simulink model "sedemo_shared_access_media"  (Simulink 7.5)
settings: Solver=VariableStepDiscrete  StartTime=0.0  StopTime=300  MaxStep=inf  RelTol=1e-3
undefined symbols (not defined in the file or in its folder): des_attributefunction_support, slcm
libraries: simeventsattributes2 x7, simeventssink1 x7, simeventsgenerators1 x5, simulink x4, simeventsrouting1 x4, simeventsqueue1 x3, simeventstranslate1 x1, simeventssignalmanage1 x1, simeventsserver1 x1
settings Model: DataTypeOverride=TrueDoubles  MinMaxOverflowLogging=ForceOff  Creator=The MathWorks Inc.  ExtModeAutoUpdateStatusClock=off
settings DataIOCC: SaveOutput=off  SaveTime=off
settings OptimizationCC: InlineInvariantSignals=on  InitFltsAndDblsToZero=on
settings DebuggingCC: AlgebraicLoopMsg=error  SaveWithParameterizedLinksMsg=none  SignalResolutionControl=TryResolveAllWithWarning  SolverPrmCheckMsg=none  InheritedTsInSrcMsg=none  DiscreteInheritContinuousMsg=none  MultiTaskDSMMsg=warning  MultiTaskCondExecSysMsg=none  StrictBusMsg=None
settings RTWCC: IncludeERTFirstTime=on
settings GRTTargetCC: TargetFcnLib=ansi_tfl_tmw.mat
settings SimEventsCC: propIdentEventSeed=12345678  propDiagAttribOutput=1  propDiagFcnCallOutput=1  propDiagStatOutput=0

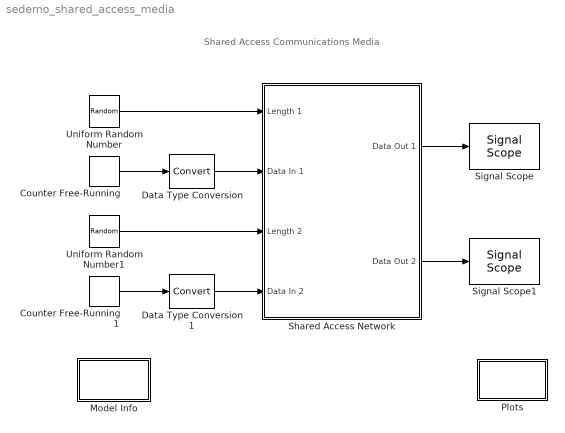
== system sedemo_shared_access_media ==
  note: Shared Access Communications Media
  Counter Free-Running : simulink/Sources/Counter Free-Running  SystemSampleTime=-1  NumBits=20  tsamp=-1
  Counter Free-Running1 : simulink/Sources/Counter Free-Running  SystemSampleTime=-1  NumBits=20  tsamp=-1
  Data Type Conversion : DataTypeConversion  OutDataType=sfix(16)  OutScaling=2^0
  Data Type Conversion1 : DataTypeConversion  OutDataType=sfix(16)  OutScaling=2^0
  Model Info : Subsystem  LoadFcn=slcm LoadBlock;  InitFcn=slcm('UpdateAllCMBlocksInThisModelInit')  mask(CMBlock){InitialSaveTempField=, InitialBlockCM=None, BlockCM=None, Frame=on, SaveTempField=, DisplayStringWithTags=Info, MaskDisplayString=Info, HorizontalTextAlignment=Center, LeftAlignmentValue=0.5, SourceBlockDiagram=sedemo_shared_access_media, TagMaxNumber=20, CMTag1=, CMTag2=, CMTag3=, CMTag4=, CMTag5=, CMTag6=, CMTag7=, CMTag8=, CMTag9=, CMTag10=, CMTag11=, CMTag12=, CMTag13=, CMTag14=, CMTag15=, CMTag16=, CMTag17=, CMTag18=, CMTag19=, CMTag20=}
      mask help: This block allows revision control information to be displayed within the model.
      settings: CopyFcn=slcm CopyBlock;  DeleteFcn=slcm Cancel;  PostSaveFcn=slcm('UpdateAllCMBlocksInThisModel')  NameChangeFcn=slcm Rename;  OpenFcn=open_system([gcb '/Information'])
      mask Display: text(str2num(LeftAlignmentValue), 0.5, MaskDisplayString, 'HorizontalAlignment', HorizontalTextAlignment)
  Plots : Subsystem
      settings: RequestExecContextInheritance=on
  Shared Access Network : Subsystem
  Signal Scope : simeventssink1/Signal Scope  Priority=1  SystemSampleTime=-1  PlotType=Stem  InputType=Signal  NumInputs=1  AttributeNameY=Count  XInputOptionSignal=Event time  XInputOptionEntity=Event time  AttributeNameX=Count  EnableEntityOutport=on  XMin=0  XMax=10  XLimitExceededOption=Stretch axis limits  YLimitExceededOption=Stretch axis limits  AxisGrid=on  AxisLegend=off  LineDisables=""  LineColors=b  LineStyles=-  LineMarkers=.  OpenScopeAtSimStart=off  Title=Data Value at Destination 1  YLabel=Data Value  XLabel=Time  FigurePosition=[4 747 305 208]  AxisZoom=off  DataStoreOption=Limited  DataPointsLimit=10000  StatNumberArrived=Off  ShowCountPlotted=on  ShowToolbar=on
      settings: YMin=0  YMax=10
  Signal Scope1 : simeventssink1/Signal Scope  Priority=1  SystemSampleTime=-1  PlotType=Stem  InputType=Signal  NumInputs=1  AttributeNameY=Count  XInputOptionSignal=Event time  XInputOptionEntity=Event time  AttributeNameX=Count  EnableEntityOutport=on  XMin=0  XMax=10  XLimitExceededOption=Stretch axis limits  YLimitExceededOption=Stretch axis limits  AxisGrid=on  AxisLegend=off  LineDisables=""  LineColors=b  LineStyles=-  LineMarkers=.  OpenScopeAtSimStart=off  Title=Data Value at Destination 1  YLabel=Data Value  XLabel=Time  FigurePosition=[4 465 305 208]  AxisZoom=off  DataStoreOption=Limited  DataPointsLimit=10000  StatNumberArrived=Off  ShowCountPlotted=on  ShowToolbar=on
      settings: YMin=0  YMax=10
  Uniform Random Number : UniformRandomNumber  Minimum=20  Maximum=2000  Seed=12345  SampleTime=0
  Uniform Random Number1 : UniformRandomNumber  Minimum=20  Maximum=2000  Seed=234567  SampleTime=0
  wires:
  Uniform Random Number/1 -> Shared Access Network/1(Length 1)
  Counter Free-Running/1 -> Data Type Conversion/1
  Uniform Random Number1/1 -> Shared Access Network/3(Length 2)
  Counter Free-Running1/1 -> Data Type Conversion1/1
  Data Type Conversion/1 -> Shared Access Network/2(Data In 1)
  Data Type Conversion1/1 -> Shared Access Network/4(Data In 2)
  Shared Access Network/1(Data Out 1) -> Signal Scope/1
  Shared Access Network/2(Data Out 2) -> Signal Scope1/1

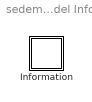
== system sedemo_shared_access_media/Model Info ==
  Information : Subsystem

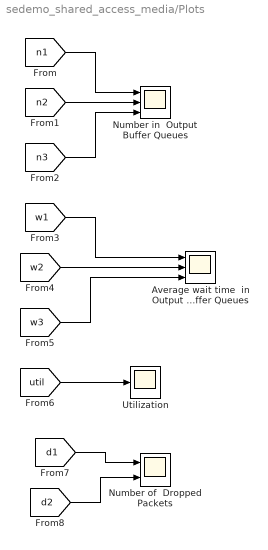
== system sedemo_shared_access_media/Plots ==
  Average wait time  in Output Buffer Queues : Scope  NumInputPorts=3
      settings: TimeRange=300  YMin=0~0~0  YMax=0.01~0.01~0.01  SaveName=ScopeData2  MaxDataPoints=10000  SampleInput=on
  Number in  Output Buffer Queues : Scope  NumInputPorts=3
      settings: TimeRange=300  YMin=0~0~0  YMax=1.5~1.5~20  MaxDataPoints=10000  SampleInput=on
  Number of  Dropped Packets : Scope  NumInputPorts=2
      settings: TimeRange=300  YMin=0~0  YMax=40~40  SaveName=ScopeData3  MaxDataPoints=10000  SampleInput=on
  Utilization : Scope
      settings: TimeRange=300  YMin=0  YMax=1.1  MaxDataPoints=10000  SampleInput=on
  wires:
  [n1] -> Number in  Output Buffer Queues/1
  [n2] -> Number in  Output Buffer Queues/2
  [n3] -> Number in  Output Buffer Queues/3
  [w1] -> Average wait time  in Output Buffer Queues/1
  [w2] -> Average wait time  in Output Buffer Queues/2
  [w3] -> Average wait time  in Output Buffer Queues/3
  [util] -> Utilization/1
  [d1] -> Number of  Dropped Packets/1
  [d2] -> Number of  Dropped Packets/2

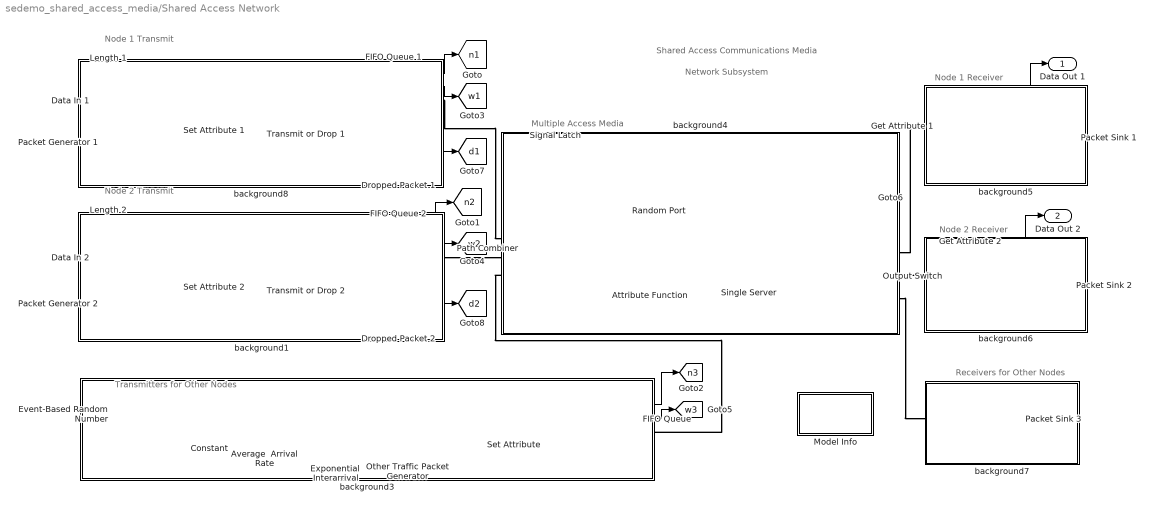
== system sedemo_shared_access_media/Shared Access Network ==
  note: Node 1 Transmit
  note: Node 2 Transmit
  note: Transmitters for Other Nodes
  note: Node 1 Receiver
  note: Node 2 Receiver
  note: Receivers for Other Nodes
  note: Shared Access Communications Media
  note: Multiple Access Media
  note: Network Subsystem
  Length 1 : Inport  OutDataType=sfix(16)  OutScaling=2^0
  Data In 1 : Inport  Port=2  OutDataType=sfix(16)  OutScaling=2^0
  Length 2 : Inport  Port=3  OutDataType=sfix(16)  OutScaling=2^0
  Data In 2 : Inport  Port=4  DataType=double  OutDataType=sfix(16)  OutScaling=2^0  OutDataTypeStr=double
  Attribute Function : Subsystem  LoadFcn=des_attributefunction_support(gcb,'LoadFcn');  StartFcn=des_attributefunction_support(gcb,'StartFcn');  mask(Attribute Function){OutputNamePrefix=out_}
      mask prompts: OutputNamePrefix "Prefix name"
      settings: CopyFcn=des_attributefunction_support(gcb,'CopyFcn');  OpenFcn=des_attributefunction_support(gcb,'OpenFcn');  ErrorFcn=des_error_redirect
      mask Display: image(des_iconLoad('attribFunction.jpg'),'center');
  Average  Arrival Rate : simulink/Math Operations/Slider Gain  SystemSampleTime=-1  low=10  gain=133.7788  high=800
  Constant : Constant  OutDataType=sfix(16)  OutScaling=2^0
  Dropped Packet 1 : simeventssink1/Entity Sink  Priority=1  SystemSampleTime=-1  AvailableForArrivals=on  StatNumberArrived=On
  Dropped Packet 2 : simeventssink1/Entity Sink  Priority=1  SystemSampleTime=-1  AvailableForArrivals=on  StatNumberArrived=On
  Event-Based Random Number : simeventsgenerators1/Signal Generators/Event-Based Random Number  SystemSampleTime=-1  distribution=Exponential  meanExp=2000  minUnif=0  maxUnif=1  pOneBern=0.25  pSuccessBino=0.5  numTrialBino=1  meanNorm=0  stdNorm=1  minTri=1  maxTri=3  modeTri=2  thresholdLogn=0  scaleLogn=1  shapeLogn=1  pSuccessGeo=0.5  meanPoiss=1  thresholdLogl=0  scaleLogl=1  thresholdGam=0  scaleGam=1  shapeGam=1  minBeta=0  maxBeta=1  shape1Beta=1  shape2Beta=1  minUnid=0  maxUnid=1  numValueUnid=2  thresholdWbl=0  scaleWbl=1  shapeWbl=1  valueVecCont=[0 1]  cdfVecCont=[0 1]  valueVecDisc=[0 1]  probVecDisc=[0.5 0.5]  seed=3669  IsProcessed=on  isConnected=1
  "Exponential  Interarrival " : Subsystem  mask(Exponential Random Number Generator){seed=0546269200}
      mask prompts: seed "Initial seed:"
      mask help: Generate random numbers with an exponential distribution. The initial seed for random number generation is specified via dialog. The input signal is used as the rate of the corresponding Poisson process.
      mask Display: plot([0.4 .13 .38 .26 .71 .44 .6 .15 .22 .5 .55 .6 .4]);
  FIFO Queue : simeventsqueue1/FIFO Queue  Priority=1  SystemSampleTime=-1  Capacity=200  EnableTOPort=off  StatNumberDeparted=Off  StatNumberInBlock=On  StatPendingEntity=Off  StatAverageWait=On  StatAverageQueueLength=Off  StatNumberTimedout=Off
  FIFO Queue 1 : simeventsqueue1/FIFO Queue  Priority=1  SystemSampleTime=-1  Capacity=1  EnableTOPort=off  StatNumberDeparted=Off  StatNumberInBlock=On  StatPendingEntity=Off  StatAverageWait=On  StatAverageQueueLength=Off  StatNumberTimedout=Off
  FIFO Queue 2 : simeventsqueue1/FIFO Queue  Priority=1  SystemSampleTime=-1  Capacity=1  EnableTOPort=off  StatNumberDeparted=Off  StatNumberInBlock=On  StatPendingEntity=Off  StatAverageWait=On  StatAverageQueueLength=Off  StatNumberTimedout=Off
  Get Attribute 1 : simeventsattributes2/Get Attribute  Priority=1  DialogController=des_ddg_create  DialogControllerArgs=DataTag11  SystemSampleTime=-1  AttributeName=Data  AttributeMissing=Error  AttributeDefaultValue=0  AttributeSendTiming=After entity departure  AttributeTreatAsVector=1  StatNumberDeparted=Off  EvaluatedDefaultAttributeValue={[]}
  Get Attribute 2 : simeventsattributes2/Get Attribute  Priority=1  DialogController=des_ddg_create  DialogControllerArgs=DataTag13  SystemSampleTime=-1  AttributeName=Data  AttributeMissing=Error  AttributeDefaultValue=0  AttributeSendTiming=After entity departure  AttributeTreatAsVector=1  StatNumberDeparted=Off  EvaluatedDefaultAttributeValue={[]}
  Model Info : Subsystem
      settings: OpenFcn=open_system([bdroot '/Model Info/Information'])
      mask Display: disp('Info')
  Other Traffic Packet Generator : simeventsgenerators1/Entity Generators/Time-Based Entity Generator  Priority=1  DialogController=des_ddg_create  DialogControllerArgs=DataTag15  SystemSampleTime=-1  GenerateEntitiesUpon=Intergeneration time from port t  Distribution=Uniform  Minimum=0  Maximum=1  Mean=1  InitialSeed=12345  Period=1  PriorityEntityGeneration=1  GenerateEntityAtSimulationStart=on  ResponseWhenBlocked=Pause generation  ResponseWhenUnblocked=Immediate restart  EntityType=Blank  StatNumberDeparted=Off  StatPendingEntity=Off  StatAverageIntergenerationTime=Off
  Output Switch : simeventsrouting1/Output Switch  Priority=1  SystemSampleTime=-1  NumberOutputPorts=3  SwitchingCriterion=From attribute  InitialSeed=34567  AttributeName=DestAddr  InitialConditionsOpt=off  InitialConditions=1  EntityBufferOpt=off  SpecifyEventPriority=off  PriorityOutputSwitchSelectPort=1  TimeoutPortOpt=off  StatNumberDeparted=Off  StatNumberTimedOut=Off  StatPendingEntity=Off  StatLastDeparturePort=Off  EvaluatedNumPorts=3
  Packet Generator 1 : simeventsgenerators1/Entity Generators/Time-Based Entity Generator  Priority=1  DialogController=des_ddg_create  DialogControllerArgs=DataTag18  SystemSampleTime=-1  GenerateEntitiesUpon=Intergeneration time from dialog  Distribution=Exponential  Minimum=0  Maximum=1  Mean=1  InitialSeed=8381  Period=1  PriorityEntityGeneration=1  GenerateEntityAtSimulationStart=on  ResponseWhenBlocked=Pause generation  ResponseWhenUnblocked=Immediate restart  EntityType=Blank  StatNumberDeparted=Off  StatPendingEntity=Off  StatAverageIntergenerationTime=Off
  Packet Generator 2 : simeventsgenerators1/Entity Generators/Time-Based Entity Generator  Priority=1  DialogController=des_ddg_create  DialogControllerArgs=DataTag20  SystemSampleTime=-1  GenerateEntitiesUpon=Intergeneration time from dialog  Distribution=Exponential  Minimum=0  Maximum=1  Mean=1  InitialSeed=4969  Period=1  PriorityEntityGeneration=1  GenerateEntityAtSimulationStart=on  ResponseWhenBlocked=Pause generation  ResponseWhenUnblocked=Immediate restart  EntityType=Blank  StatNumberDeparted=Off  StatPendingEntity=Off  StatAverageIntergenerationTime=Off
  Packet Sink 1 : simeventssink1/Entity Sink  Priority=1  SystemSampleTime=-1  AvailableForArrivals=on  StatNumberArrived=Off
  Packet Sink 2 : simeventssink1/Entity Sink  Priority=1  SystemSampleTime=-1  AvailableForArrivals=on  StatNumberArrived=Off
  Packet Sink 3 : simeventssink1/Entity Sink  Priority=1  SystemSampleTime=-1  AvailableForArrivals=on  StatNumberArrived=Off
  Path Combiner : simeventsrouting1/Path Combiner  Priority=1  SystemSampleTime=-1  NumberInputPorts=3  InputPortPrecedence=From signal port p  InitialSeed=45675  SpecifyEventPriority=off  PriorityPathCombinerPortPrecedenceSelection=4100  StatNumberDeparted=On  StatLastArrivalPort=Off  EvaluatedNumPorts=3
  Random Port : simeventsgenerators1/Signal Generators/Event-Based Random Number  SystemSampleTime=-1  distribution=Arbitrary discrete  meanExp=2000  minUnif=0  maxUnif=1  pOneBern=0.25  pSuccessBino=0.5  numTrialBino=1  meanNorm=0  stdNorm=1  minTri=1  maxTri=3  modeTri=2  thresholdLogn=0  scaleLogn=1  shapeLogn=1  pSuccessGeo=0.5  meanPoiss=1  thresholdLogl=0  scaleLogl=1  thresholdGam=0  scaleGam=1  shapeGam=1  minBeta=0  maxBeta=1  shape1Beta=1  shape2Beta=1  minUnid=0  maxUnid=1  numValueUnid=2  thresholdWbl=0  scaleWbl=1  shapeWbl=1  valueVecCont=[0 1]  cdfVecCont=[0 1]  valueVecDisc=[1 2 3]  probVecDisc=[0.005 0.005 0.990]  seed=2255  IsProcessed=on  isConnected=1
  Set Attribute : simeventsattributes2/Set Attribute  Priority=1  DialogController=des_ddg_create  DialogControllerArgs=DataTag26  SystemSampleTime=-1  AttributeFrom=Dialog|Signal port|Dialog|Dialog  AttributeName=DestAddr|Length|Data|DataRate  AttributeTreatAsVector=1|1|1|1  AttributeValue=3|0|0|1000000  AttributeCreate=on  StatNumberDeparted=Off  EvaluatedAttributeValue={3;[];0;1000000}
  Set Attribute 1 : simeventsattributes2/Set Attribute  Priority=1  DialogController=des_ddg_create  DialogControllerArgs=DataTag28  SystemSampleTime=-1  AttributeFrom=Dialog|Signal port|Signal port|Dialog  AttributeName=DestAddr|Length|Data|DataRate  AttributeTreatAsVector=1|1|1|1  AttributeValue=2|0|0|1000000  AttributeCreate=on  StatNumberDeparted=Off  EvaluatedAttributeValue={2;[];[];1000000}
  Set Attribute 2 : simeventsattributes2/Set Attribute  Priority=1  DialogController=des_ddg_create  DialogControllerArgs=DataTag30  SystemSampleTime=-1  AttributeFrom=Dialog|Signal port|Signal port|Dialog  AttributeName=DestAddr|Length|Data|DataRate  AttributeTreatAsVector=1|1|1|1  AttributeValue=1|0|0|1000000  AttributeCreate=on  StatNumberDeparted=Off  EvaluatedAttributeValue={1;[];[];1000000}
  Signal Latch : simeventssignalmanage1/Signal Latch  Priority=1  SystemSampleTime=-1  InitialMemoryValue=1  WriteMemoryUpon=Change in signal from port wvc  MemoryWriteEdgeOption=Rising  SpecifyWriteEventPriority=on  PriorityMemoryWrite=7100  ReadMemoryUpon=Write to memory event  MemoryReadEdgeOption=Falling  SpecifyReadEventPriority=on  PriorityMemoryRead=7000  ReportMemoryState=off  ReportMemoryUponWrite=off  ReportMemoryUponRead=on
  Single Server : simeventsserver1/Single Server  Priority=1  SystemSampleTime=-1  ServiceTimeFrom=Attribute  ServiceTime=1  AttributeName=ServiceTime  PriorityServiceCompletion=500  PermitPreemption=off  SortingAttributeName=PriorityAttributeName  SortingDirection=Ascending  WriteToAttribute=off  ResidualAttributeName=ResidualServiceTime  CreateAttribute=on  EnableTOPort=off  StatNumberDeparted=Off  StatNumberInBlock=Off  StatNumberPreempted=Off  StatPendingEntity=Off  StatAverageWait=Off  StatUtilization=On  StatNumberTimedout=Off
  Transmit or Drop 1 : simeventsrouting1/Output Switch  Priority=1  SystemSampleTime=-1  NumberOutputPorts=2  SwitchingCriterion=First port that is not blocked  InitialSeed=34567  AttributeName=Attribute1  InitialConditionsOpt=off  InitialConditions=1  EntityBufferOpt=off  SpecifyEventPriority=off  PriorityOutputSwitchSelectPort=1  TimeoutPortOpt=off  StatNumberDeparted=Off  StatNumberTimedOut=Off  StatPendingEntity=Off  StatLastDeparturePort=Off  EvaluatedNumPorts=2
  Transmit or Drop 2 : simeventsrouting1/Output Switch  Priority=1  SystemSampleTime=-1  NumberOutputPorts=2  SwitchingCriterion=First port that is not blocked  InitialSeed=34567  AttributeName=Attribute1  InitialConditionsOpt=off  InitialConditions=1  EntityBufferOpt=off  SpecifyEventPriority=off  PriorityOutputSwitchSelectPort=1  TimeoutPortOpt=off  StatNumberDeparted=Off  StatNumberTimedOut=Off  StatPendingEntity=Off  StatLastDeparturePort=Off  EvaluatedNumPorts=2
  background1 : Subsystem
      mask Display: disp('')
  background3 : Subsystem
      mask Display: disp('')
  background4 : Subsystem
      mask Display: disp('')
  background5 : Subsystem
      mask Display: disp('')
  background6 : Subsystem
      mask Display: disp('')
  background7 : Subsystem
      mask Display: disp('')
  background8 : Subsystem
      mask Display: disp('')
  Data Out 1 : Outport  OutDataType=sfix(16)  OutScaling=2^0
  Data Out 2 : Outport  Port=2  OutDataType=sfix(16)  OutScaling=2^0
  tag scope: d1=global, d2=global, n1=global, n2=global, n3=global, util=global, w1=global, w2=global, w3=global
  wires:
  FIFO Queue 1/1 -> [n1]
  Length 1/1 -> Set Attribute 1/1
  FIFO Queue 1/2 -> [w1]
  Data In 1/1 -> Set Attribute 1/2
  Get Attribute 1/1 -> Data Out 1/1
  Length 2/1 -> Set Attribute 2/1
  Single Server/1 -> [util]
  Get Attribute 2/1 -> Data Out 2/1
  Data In 2/1 -> Set Attribute 2/2
  FIFO Queue/1 -> [n3]
  FIFO Queue/2 -> [w3]
  Event-Based Random Number/1 -> Set Attribute/1
  Dropped Packet 1/1 -> [d1]
  Dropped Packet 2/1 -> [d2]
  Constant/1 -> Average  Arrival Rate/1
  Average  Arrival Rate/1 -> "Exponential  Interarrival "/1(rate)
  "Exponential  Interarrival "/1(Out1) -> Other Traffic Packet Generator/1
  FIFO Queue 2/2 -> [w2]
  FIFO Queue 2/1 -> [n2]
  Signal Latch/1 -> Path Combiner/1
  Random Port/1 -> Signal Latch/2
  Path Combiner/1 -> Signal Latch/1
  connections:
  Single Server/RConn1 -- Output Switch/LConn1
  Attribute Function/LConn1 -- Path Combiner/RConn1
  Output Switch/RConn1 -- Get Attribute 1/LConn1
  Get Attribute 1/RConn1 -- Packet Sink 1/LConn1
  Get Attribute 2/LConn1 -- Output Switch/RConn2
  Get Attribute 2/RConn1 -- Packet Sink 2/LConn1
  Other Traffic Packet Generator/RConn1 -- Set Attribute/LConn1
  Set Attribute/RConn1 -- FIFO Queue/LConn1
  FIFO Queue 1/RConn1 -- Path Combiner/LConn1
  FIFO Queue 2/RConn1 -- Path Combiner/LConn2
  Output Switch/RConn3 -- Packet Sink 3/LConn1
  Path Combiner/LConn3 -- FIFO Queue/RConn1
  Packet Generator 1/RConn1 -- Set Attribute 1/LConn1
  Packet Generator 2/RConn1 -- Set Attribute 2/LConn1
  Transmit or Drop 1/LConn1 -- Set Attribute 1/RConn1
  FIFO Queue 1/LConn1 -- Transmit or Drop 1/RConn1
  Transmit or Drop 1/RConn2 -- Dropped Packet 1/LConn1
  Transmit or Drop 2/RConn2 -- Dropped Packet 2/LConn1
  Set Attribute 2/RConn1 -- Transmit or Drop 2/LConn1
  Transmit or Drop 2/RConn1 -- FIFO Queue 2/LConn1
  Attribute Function/RConn1 -- Single Server/LConn1

== system sedemo_shared_access_media/Model Info/Information ==
  note: Shared Access Communications Media
  note: This model is an abstraction of a communications bus or shared media. Each
      | transmitter that uses the bus has exclusive access until the use is completed.
      | In this model, transmit node 1 is sending to receive node 2, and vice versa.
      | Background traffic from other nodes in the network is modeled in the aggregate.
      | You can adjust the aggregate traffic for the other nodes using a slider in
      | the Avg. Arrival Rate block.
      |
      | Using the plots, you can monitor bus/media utilization, queue lengths, average
      | waiting times, and the number of dropped packets.
      |
      | The bus/media abstraction is enclosed in a subsystem to facilitate copying into
      | another model. For example, you can explore further by modeling the delays
      | incurred over a bus between two processors.

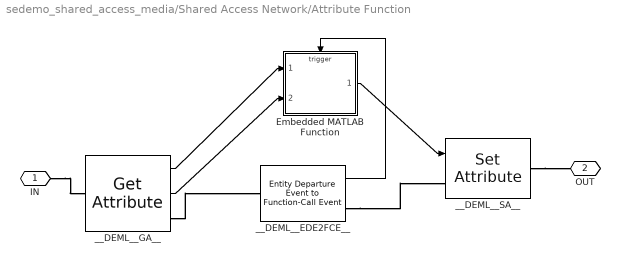
== system sedemo_shared_access_media/Shared Access Network/Attribute Function ==
  Embedded MATLAB Function : Stateflow chart  TreatAsAtomicUnit=on
      settings: PropExecContextOutsideSubsystem=on
  __DEML__EDE2FCE__ : simeventstranslate1/Entity Departure Event to Function-Call Event  Priority=1  SystemSampleTime=-1  TimingFunctionCallF1=Before entity departure  EnableE1Port=off  EnableF2Port=off  TimingFunctionCallF2=Before entity departure  EnableE2Port=off  StatNumberDeparted=Off  StatNumberF1Calls=Off  StatNumberF2Calls=Off  IsInsideAFB=on
  __DEML__GA__ : simeventsattributes2/Get Attribute  Priority=1  DialogController=des_ddg_create  DialogControllerArgs=DataTag2  SystemSampleTime=-1  AttributeName=Length|DataRate  AttributeMissing=Error|Error  AttributeDefaultValue=1|1  AttributeSendTiming=Before entity departure|Before entity departure  AttributeTreatAsVector=1|1  StatNumberDeparted=Off  EvaluatedDefaultAttributeValue={[];[]}
  __DEML__SA__ : simeventsattributes2/Set Attribute  Priority=1  DialogController=des_ddg_create  DialogControllerArgs=DataTag4  SystemSampleTime=-1  AttributeFrom=Signal port  AttributeName=ServiceTime  AttributeTreatAsVector=1  AttributeValue=1  AttributeCreate=on  StatNumberDeparted=Off  EvaluatedAttributeValue={[]}
  IN : PMIOPort  Port=1  Side=Left
  OUT : PMIOPort  Port=2  Side=Right
  wires:
  __DEML__EDE2FCE__/1 -> Embedded MATLAB Function/Trigger
  __DEML__GA__/1 -> Embedded MATLAB Function/1(Length)
  __DEML__GA__/2 -> Embedded MATLAB Function/2(DataRate)
  Embedded MATLAB Function/1(out_ServiceTime) -> __DEML__SA__/1
  connections:
  __DEML__SA__/RConn1 -- OUT/RConn1
  IN/RConn1 -- __DEML__GA__/LConn1
  __DEML__GA__/RConn1 -- __DEML__EDE2FCE__/LConn1
  __DEML__EDE2FCE__/RConn1 -- __DEML__SA__/LConn1

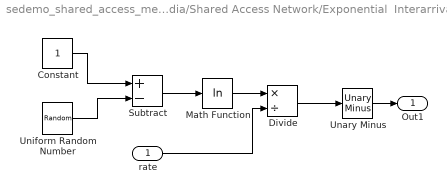
== system sedemo_shared_access_media/Shared Access Network/Exponential  Interarrival  ==
  rate : Inport  OutDataType=sfix(16)  OutScaling=2^0
  Constant : Constant  OutDataType=sfix(16)  OutScaling=2^0
  Divide : Product  Inputs=*/  OutDataType=sfix(16)  OutScaling=2^-10
  Math Function : Math  Operator=log  OutDataType=sfix(16)  OutScaling=2^0  SaturateOnIntegerOverflow=on
  Subtract : Sum  Inputs=+-  OutDataType=sfix(16)  OutScaling=2^-10
  Unary Minus : simulink/Math Operations/Unary Minus  DoSatur=off
  Uniform Random Number : UniformRandomNumber  Minimum=0  Seed=seed  SampleTime=0
  Out1 : Outport  OutDataType=sfix(16)  OutScaling=2^0
  wires:
  Unary Minus/1 -> Out1/1
  Divide/1 -> Unary Minus/1
  Subtract/1 -> Math Function/1
  Uniform Random Number/1 -> Subtract/2
  Constant/1 -> Subtract/1
  rate/1 -> Divide/2
  Math Function/1 -> Divide/1

== system sedemo_shared_access_media/Shared Access Network/Model Info ==

== system sedemo_shared_access_media/Shared Access Network/background1 ==

== system sedemo_shared_access_media/Shared Access Network/background3 ==

== system sedemo_shared_access_media/Shared Access Network/background4 ==

== system sedemo_shared_access_media/Shared Access Network/background5 ==

== system sedemo_shared_access_media/Shared Access Network/background6 ==

== system sedemo_shared_access_media/Shared Access Network/background7 ==

== system sedemo_shared_access_media/Shared Access Network/background8 ==

== matlab function Shared Access Network/Attribute Function/Embedded MATLAB Function ==
  data: Length input double; out_ServiceTime output double; DataRate input double
  events: trigger input FUNCTION_CALL_EVENT
function out_ServiceTime  = fcn(Length,DataRate)

out_ServiceTime = divide(numerictype(Length),Length,DataRate);
